simulink model "Fig51"  (R2014b)
settings: Solver=ode3  StartTime=0.0  StopTime=.05  FixedStep=2e-3  RelTol=1e-3
libraries: commrandsrc2 x2, commutil2 x1
settings Model: Creator=Silage  LastModifiedBy=Silage

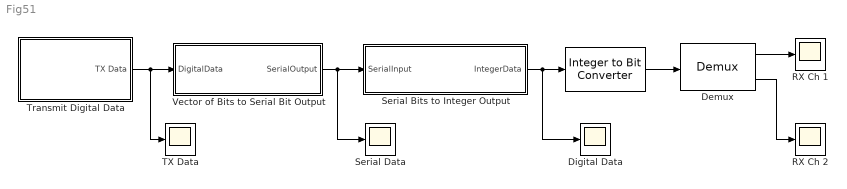
== system Fig51 ==
  " " : commutil2/Integer to Bit Converter  nbits=2  signedInputValues=Unsigned  bitOrder=LSB first  outDtype=Inherit via internal rule
  Demux : Demux  Outputs=2
  Digital Data : Scope
      settings: SaveName=ScopeData6
  RX Ch 1 : Scope
      settings: YMin=-1  YMax=2
  RX Ch 2 : Scope
  Serial Bits to Integer Output : MATLAB Function  TreatAsAtomicUnit=on
  Serial Data : Scope
      settings: SaveName=ScopeData3
  TX Data : Scope
      settings: SaveName=ScopeData2
  Transmit Digital Data : Subsystem
  Vector of Bits to Serial Bit Output : MATLAB Function  TreatAsAtomicUnit=on
  wires:
  Demux/1 -> RX Ch 1/1
  Demux/2 -> RX Ch 2/1
  Vector of Bits to Serial Bit Output/1(SerialOutput) -> Serial Bits to Integer Output/1(SerialInput), Serial Data/1
  Serial Bits to Integer Output/1(IntegerData) -> " "/1, Digital Data/1
  " "/1 -> Demux/1
  Transmit Digital Data/1(TX Data) -> Vector of Bits to Serial Bit Output/1(DigitalData), TX Data/1

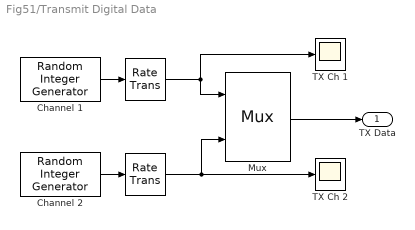
== system Fig51/Transmit Digital Data ==
  " " : RateTransition  OutPortSampleTime=2e-3
  "  " : RateTransition  OutPortSampleTime=2e-3
  Channel 1 : commrandsrc2/Random Integer Generator  mul=2  seed=37  Ts=4e-3  frameBased=off  sampPerFrame=1  orient=on  outDataType=double
  Channel 2 : commrandsrc2/Random Integer Generator  mul=2  seed=59  Ts=4e-3  frameBased=off  sampPerFrame=1  orient=on  outDataType=double
  Mux : Mux  Inputs=2
      settings: DisplayOption=signals
  TX Ch 1 : Scope
      settings: SaveName=ScopeData4
  TX Ch 2 : Scope
      settings: SaveName=ScopeData5
  TX Data : Outport
  wires:
  Mux/1 -> TX Data/1
  Channel 1/1 -> " "/1
  " "/1 -> Mux/1, TX Ch 1/1
  Channel 2/1 -> "  "/1
  "  "/1 -> TX Ch 2/1, Mux/2

== matlab function Fig51/Serial Bits to Integer Output ==
  data: SerialInput input; IntegerData output
function IntegerData = fcn(SerialInput)
%#codegen

persistent SmpDat  SmpNum SmpDatOld

if isempty(SmpNum)
    SmpNum = 0;
    SmpDat = 0;
    SmpDatOld = 0;
    IntegerData = 0; %#ok<*NASGU>
end

SmpNum = SmpNum + 1;
if (SmpNum == 3)
    SmpNum = 1;
    SmpDatOld = SmpDat;
    IntegerData = SmpDatOld;
    SmpDat = SerialInput;    
else
    IntegerData = SmpDatOld;
    SmpDat = SmpDat + SerialInput*2^(SmpNum - 1);
end

end

== matlab function Fig51/Vector of Bits to Serial Bit Output ==
  data: DigitalData input; SerialOutput output
function SerialOutput = fcn(DigitalData)
%#codegen
persistent SmpDat SmpNum

if isempty(SmpNum)
    SmpNum = 1;
    SmpDat = DigitalData;
end

SmpDat = DigitalData;
SerialOutput = SmpDat(SmpNum);
SmpNum = SmpNum + 1;
if (SmpNum == 3)
    SmpNum = 1;
end

end
